simulink subsystem "solution"  (R2024a)
settings: Solver=VariableStepAuto  StartTime=0.0  StopTime=10.0  RelTol=1e-3
settings Model: Creator=ngcoya  LastModifiedBy=ngcoya

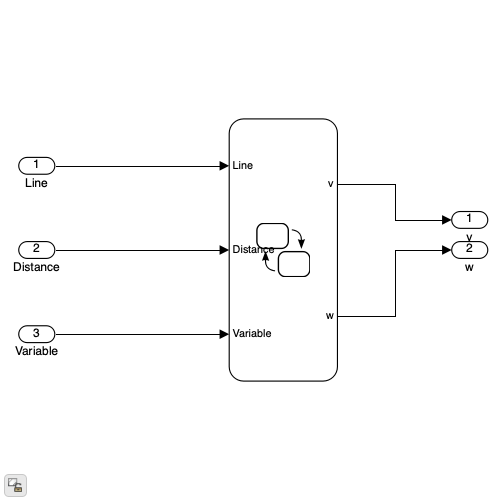
[thumbnail: Simulink's stored preview of the top-level diagram]
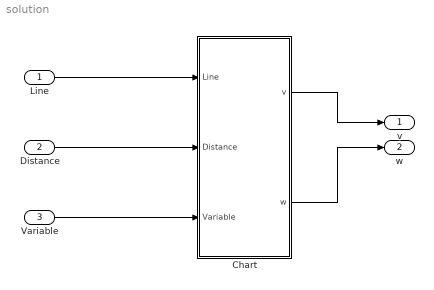
== system solution ==
  Line : Inport  PortDimensions=2
  Distance : Inport  Port=2  PortDimensions=3
  Variable : Inport  Port=3  PortDimensions=2
  Chart : Stateflow chart  TreatAsAtomicUnit=on
  v : Outport
  w : Outport  Port=2
  wires:
  Chart/2(w) -> w/1
  Line/1 -> Chart/1(Line)
  Chart/1(v) -> v/1
  Variable/1 -> Chart/3(Variable)
  Distance/1 -> Chart/2(Distance)

== stateflow chart solution/Chart ==
  data: Line input; v output; Distance input; Variable input; w output; theta local
